simulink model "simulink_ft_fault_injection"  (R2017b)
settings: Solver=FixedStepAuto  StartTime=0.0  StopTime=Tend  FixedStep=hp  RelTol=1e-3
undefined symbols (not defined in the file): actuation_delay, Ad_plant, Bd_plant, Cd_plant, controller_mode, Dd_plant, delay_length, error_probability, f, F1, F2, F3, hp, K1, K2, K3, mode_switching_enable, n, ref, ref_array, ref_sampling_factor, Sat_u, Sm
settings Model: SimulationMode=accelerator  SnapshotInterval=2  Creator=juan  LastModifiedBy=jvalencia
settings CodeAppCC: StateflowObjectComments=on

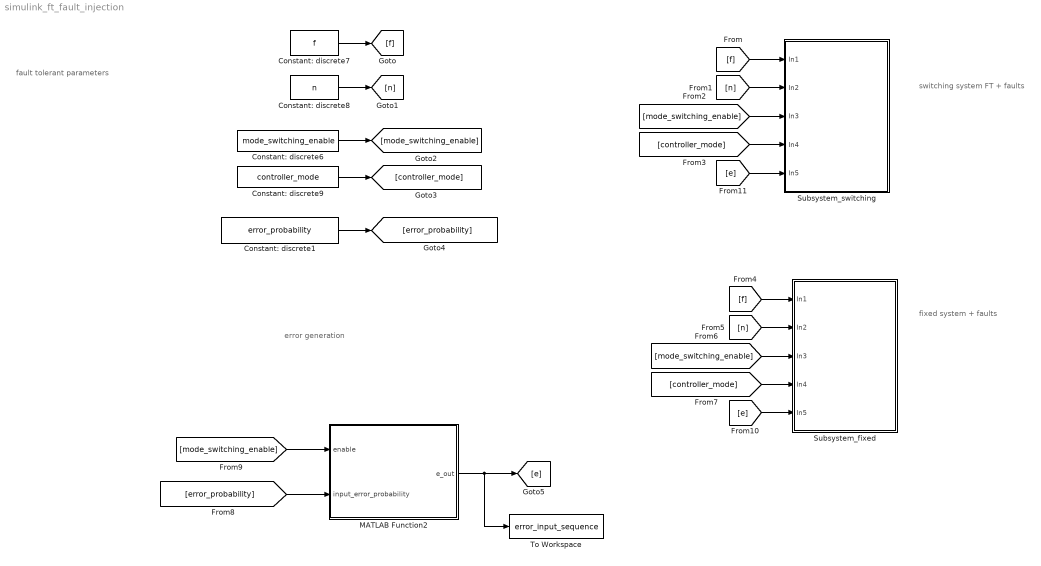
== system simulink_ft_fault_injection ==
  note: fault tolerant parameters
  note: fixed system + faults
  note: switching system FT + faults
  note: error generation
  Constant: discrete1 : Constant  Value=error_probability  SampleTime=Sm
  Constant: discrete6 : Constant  Value=mode_switching_enable  SampleTime=Sm
  Constant: discrete7 : Constant  Value=f  OutDataTypeStr=single  SampleTime=Sm
  Constant: discrete8 : Constant  Value=n  OutDataTypeStr=single  SampleTime=Sm
  Constant: discrete9 : Constant  Value=controller_mode  SampleTime=Sm
  MATLAB Function2 : MATLAB Function  TreatAsAtomicUnit=on  SystemSampleTime=Sm
  Subsystem_fixed : Subsystem
  Subsystem_switching : Subsystem
  To Workspace : ToWorkspace  VariableName=error_input_sequence  SaveFormat=Timeseries  SampleTime=Sm
  wires:
  Constant: discrete7/1 -> [f]
  Constant: discrete8/1 -> [n]
  Constant: discrete6/1 -> [mode_switching_enable]
  Constant: discrete9/1 -> [controller_mode]
  [f] -> Subsystem_switching/1(In1)
  [n] -> Subsystem_switching/2(In2)
  [mode_switching_enable] -> Subsystem_switching/3(In3)
  [controller_mode] -> Subsystem_switching/4(In4)
  Constant: discrete1/1 -> [error_probability]
  [mode_switching_enable] -> MATLAB Function2/1(enable)
  [error_probability] -> MATLAB Function2/2(input_error_probability)
  [f] -> Subsystem_fixed/1(In1)
  [n] -> Subsystem_fixed/2(In2)
  [mode_switching_enable] -> Subsystem_fixed/3(In3)
  [controller_mode] -> Subsystem_fixed/4(In4)
  MATLAB Function2/1(e_out) -> To Workspace/1, [e]
  [e] -> Subsystem_fixed/5(In5)
  [e] -> Subsystem_switching/5(In5)

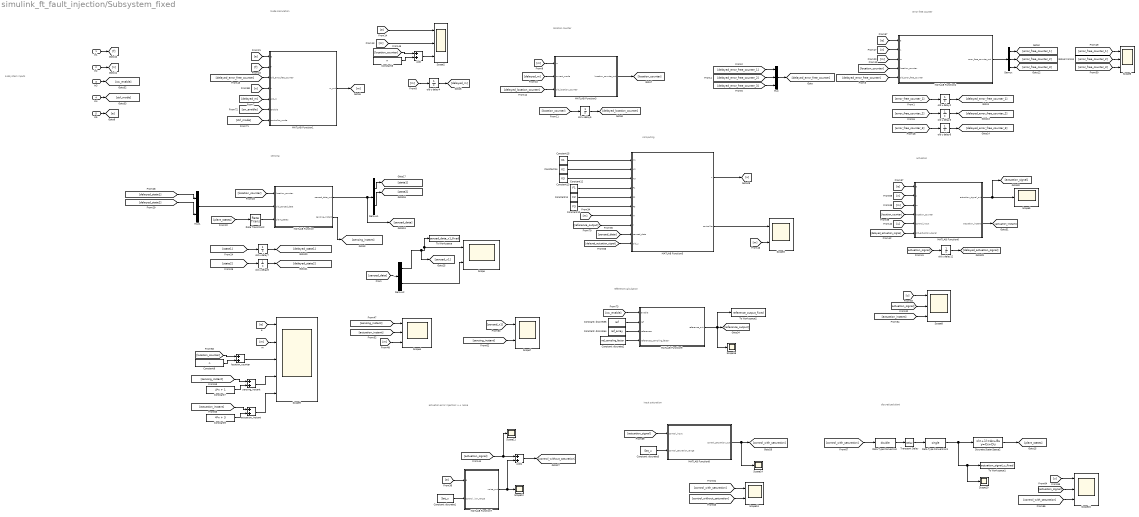
== system simulink_ft_fault_injection/Subsystem_fixed ==
  note: mode calculation
  note: location
      | counter
  note: error free counter
  note: sensing
  note: computing
  note: actuation
  note: actuation error injection: u + noise
  note: discretized plant
  note: input saturation
  note: reference calculation
  note: subsystem inputs
  In1 : Inport
  In2 : Inport  Port=2
  In3 : Inport  Port=3
  In4 : Inport  Port=4
  In5 : Inport  Port=5
  Add : Sum
  Add1 : Sum
  Constant10 : Constant  Value=F3  OutDataTypeStr=single  SampleTime=Sm
  Constant11 : Constant  Value=F2  OutDataTypeStr=single  SampleTime=Sm
  Constant12 : Constant  Value=F1  OutDataTypeStr=single  SampleTime=Sm
  Constant13 : Constant  Value=K3  OutDataTypeStr=single  SampleTime=Sm
  Constant14 : Constant  Value=K2  OutDataTypeStr=single  SampleTime=Sm
  Constant15 : Constant  Value=K1  OutDataTypeStr=single  SampleTime=Sm
  Constant6 : Constant  Value=n  SampleTime=Sm
  Constant7 : Constant  Value=4*n + 1  SampleTime=Sm
  Constant8 : Constant  Value=n  SampleTime=Sm
  Constant9 : Constant  Value=4*n + 3  SampleTime=Sm
  Constant: discrete1 : Constant  Value=Sat_u  OutDataTypeStr=single  SampleTime=Sm
  Constant: discrete2 : Constant  Value=ref_sampling_factor  OutDataTypeStr=single  SampleTime=Sm
  Constant: discrete3 : Constant  Value=Sat_u  OutDataTypeStr=single  SampleTime=Sm
  Constant: discrete4 : Constant  Value=ref_array  OutDataTypeStr=single  SampleTime=Sm
  Constant: discrete5 : Constant  Value=ref  OutDataTypeStr=single  SampleTime=Sm
  Data Type Conversion : DataTypeConversion  OutDataTypeStr=double
  Data Type Conversion1 : DataTypeConversion  OutDataTypeStr=single
  Demux : Demux  Outputs=3
  Demux1 : Demux  Outputs=2
  Demux2 : Demux  Outputs=2
  Discrete State-Space2 : DiscreteStateSpace  A=Ad_plant  B=Bd_plant  C=Cd_plant  D=Dd_plant  SampleTime=hp
  MATLAB Function : MATLAB Function  TreatAsAtomicUnit=on
  MATLAB Function1 : MATLAB Function  TreatAsAtomicUnit=on
  MATLAB Function3 : MATLAB Function  TreatAsAtomicUnit=on  SystemSampleTime=Sm
  MATLAB Function4 : MATLAB Function  TreatAsAtomicUnit=on  SystemSampleTime=Sm
  MATLAB Function5 : MATLAB Function  TreatAsAtomicUnit=on
  MATLAB Function6 : MATLAB Function  TreatAsAtomicUnit=on
  MATLAB Function7 : MATLAB Function  TreatAsAtomicUnit=on
  MATLAB Function8 : MATLAB Function  TreatAsAtomicUnit=on
  MATLAB Function9 : MATLAB Function  TreatAsAtomicUnit=on
  Mux : Mux  Inputs=3
  Mux1 : Mux  Inputs=2
  Rate Transition2 : RateTransition  OutPortSampleTime=Sm
  Scope{,3,7,13} (4 alike) : Scope  NumInputPorts=2
  Scope{5,10..12,14,16} (6 alike) : Scope
  Scope{2,4,6,8,15} (5 alike) : Scope  NumInputPorts=3
  Scope9 : Scope  NumInputPorts=5
  To Workspace : ToWorkspace  VariableName=sensed_data_x1_fixed  SaveFormat=Timeseries  SampleTime=Sm
  To Workspace1 : ToWorkspace  VariableName=actuation_signal_u_fixed  SaveFormat=Timeseries  SampleTime=Sm
  To Workspace2 : ToWorkspace  VariableName=reference_output_fixed  SaveFormat=Timeseries  SampleTime=Sm
  Transport Delay : TransportDelay  DelayTime=actuation_delay
  actuation_instant : Sum
  location_counter : Sum
  old u delay{2..8,12} (8 alike) : UnitDelay  SampleTime=Sm
  sensing_instant : Sum
  wires:
  [state2] -> old u delay8/1
  Constant14/1 -> MATLAB Function5/2(K2)
  Constant15/1 -> MATLAB Function5/1(K1)
  [reference_output] -> MATLAB Function5/8(r)
  [actuation_signal] -> Scope8/2
  [u] -> Scope8/1
  [e] -> MATLAB Function4/1(e)
  location_counter/1 -> Scope9/3
  [m] -> MATLAB Function5/7(m)
  Constant10/1 -> MATLAB Function5/6(F3)
  Constant11/1 -> MATLAB Function5/5(F2)
  Constant12/1 -> MATLAB Function5/4(F1)
  [actuation_instant] -> Scope8/3
  Demux2/1 -> [sensed_x1], To Workspace/1, Scope/1
  [e] -> MATLAB Function6/1(e)
  actuation_instant/1 -> Scope9/5
  [delayed_actuation_signal] -> MATLAB Function5/10(old_u)
  [sensed_data] -> MATLAB Function5/9(sensed_data)
  Constant13/1 -> MATLAB Function5/3(K3)
  [n] -> MATLAB Function6/2(n)
  [sensed_x1] -> Scope7/1
  Transport Delay/1 -> Data Type Conversion1/1
  [actuation_signal] -> Add1/1, Scope11/1
  MATLAB Function6/1(actuation_signal_out) -> [actuation_signal], Scope5/1
  [sensing_instant] -> Scope7/2
  Constant: discrete1/1 -> MATLAB Function7/2(control_saturation_range)
  Add1/1 -> [control_without_saturation]
  Constant: discrete3/1 -> MATLAB Function8/2(control_saturation_range)
  Data Type Conversion/1 -> Transport Delay/1
  [control_with_saturation] -> Scope13/1
  [e] -> Scope9/1
  [control_without_saturation] -> Scope13/2
  MATLAB Function8/1(control_saturation_out) -> Scope14/1, [control_with_saturation]
  [actuation_signal] -> Scope15/2
  [u] -> Scope15/1
  [control_with_saturation] -> Scope15/3
  [actuation_signal] -> MATLAB Function8/1(control_input)
  [control_with_saturation] -> Data Type Conversion/1
  [sw_enable] -> MATLAB Function1/6(enable)
  Constant: discrete4/1 -> MATLAB Function9/3(references)
  Constant: discrete5/1 -> MATLAB Function9/2(ref)
  [sw_enable] -> MATLAB Function9/1(enable)
  Constant: discrete2/1 -> MATLAB Function9/4(references_sampling_factor)
  MATLAB Function9/1(reference_out) -> To Workspace2/1, Scope16/1, [reference_output]
  Data Type Conversion1/1 -> Discrete State-Space2/1, Scope10/1, To Workspace1/1
  MATLAB Function7/1(noise_out) -> Scope12/1, Add1/2
  [e] -> MATLAB Function7/1(e)
  old u delay8/1 -> [delayed_state2]
  [state1] -> old u delay7/1
  [location_counter] -> MATLAB Function6/4(location_counter)
  Demux2/2 -> Scope/2
  [e] -> MATLAB Function1/1(e)
  [delayed_error_free_counter] -> MATLAB Function4/5(old_error_free_counter)
  [delayed_error_free_counter] -> MATLAB Function1/3(old_error_free_counter)
  Mux/1 -> [delayed_error_free_counter]
  MATLAB Function5/1(u) -> [u]
  [error_free_counter_3] -> Scope6/3
  Constant7/1 -> sensing_instant/2
  MATLAB Function5/2(controller) -> Scope3/1
  [actuation_instant] -> actuation_instant/1
  [location_counter] -> location_counter/1
  Constant9/1 -> actuation_instant/2
  [sensing_instant] -> sensing_instant/1
  [actuation_instant] -> Scope4/2
  [m] -> Scope4/3
  MATLAB Function6/2(actuation_instant) -> [actuation_instant]
  Constant8/1 -> location_counter/2
  [sensing_instant] -> Scope4/1
  [m] -> Scope9/2
  MATLAB Function/2(sensing_instant) -> [sensing_instant]
  [m] -> Scope3/2
  [error_free_counter_2] -> Scope6/2
  [error_free_counter_1] -> Scope6/1
  Add/1 -> Scope2/3
  Constant6/1 -> Add/2
  [location_counter] -> Add/1
  [delayed_state2] -> Mux1/2
  [actuation_signal] -> old u delay12/1
  [delayed_state1] -> Mux1/1
  old u delay12/1 -> [delayed_actuation_signal]
  [delayed_actuation_signal] -> MATLAB Function6/6(old_actuation_signal)
  [sensed_data] -> Demux2/1
  sensing_instant/1 -> Scope9/4
  Mux1/1 -> MATLAB Function/2(old_sensed_data)
  old u delay7/1 -> [delayed_state1]
  Rate Transition2/1 -> MATLAB Function/3(plant_states)
  [m] -> MATLAB Function6/3(m)
  [u] -> MATLAB Function6/5(control_input)
  old u delay2/1 -> [delayed_error_free_counter_1]
  [location_counter] -> old u delay5/1
  [plant_states] -> Rate Transition2/1
  [delayed_error_free_counter_3] -> Mux/3
  [m] -> MATLAB Function3/1(m)
  [n] -> MATLAB Function4/2(n)
  Demux/3 -> [error_free_counter_3]
  old u delay4/1 -> [delayed_m]
  [error_free_counter_1] -> old u delay2/1
  MATLAB Function1/1(m_out) -> [m]
  old u delay3/1 -> [delayed_error_free_counter_2]
  old u delay6/1 -> [delayed_error_free_counter_3]
  MATLAB Function/1(sensed_data_out) -> [sensed_data], Demux1/1
  Demux1/2 -> [state2]
  [delayed_error_free_counter_1] -> Mux/1
  [m] -> MATLAB Function4/3(m)
  Discrete State-Space2/1 -> [plant_states]
  Demux/2 -> [error_free_counter_2]
  [delayed_error_free_counter_2] -> Mux/2
  [delayed_m] -> MATLAB Function3/2(current_mode)
  MATLAB Function3/1(location_counter_out) -> [location_counter]
  [delayed_location_counter] -> MATLAB Function3/3(old_location_counter)
  old u delay5/1 -> [delayed_location_counter]
  Demux/1 -> [error_free_counter_1]
  Demux1/1 -> [state1]
  [m] -> old u delay4/1
  [location_counter] -> MATLAB Function4/4(location_counter)
  [e] -> Scope2/1
  [m] -> Scope2/2
  [error_free_counter_2] -> old u delay3/1
  [delayed_m] -> MATLAB Function1/5(old_m)
  [error_free_counter_3] -> old u delay6/1
  MATLAB Function4/1(error_free_counter_out) -> Demux/1
  [location_counter] -> MATLAB Function/1(location_counter)
  [ctrl_mode] -> MATLAB Function1/7(controller_mode)
  [f] -> MATLAB Function1/2(f)
  [n] -> MATLAB Function1/4(n)
  In1/1 -> [f]
  In2/1 -> [n]
  In3/1 -> [sw_enable]
  In4/1 -> [ctrl_mode]
  In5/1 -> [e]

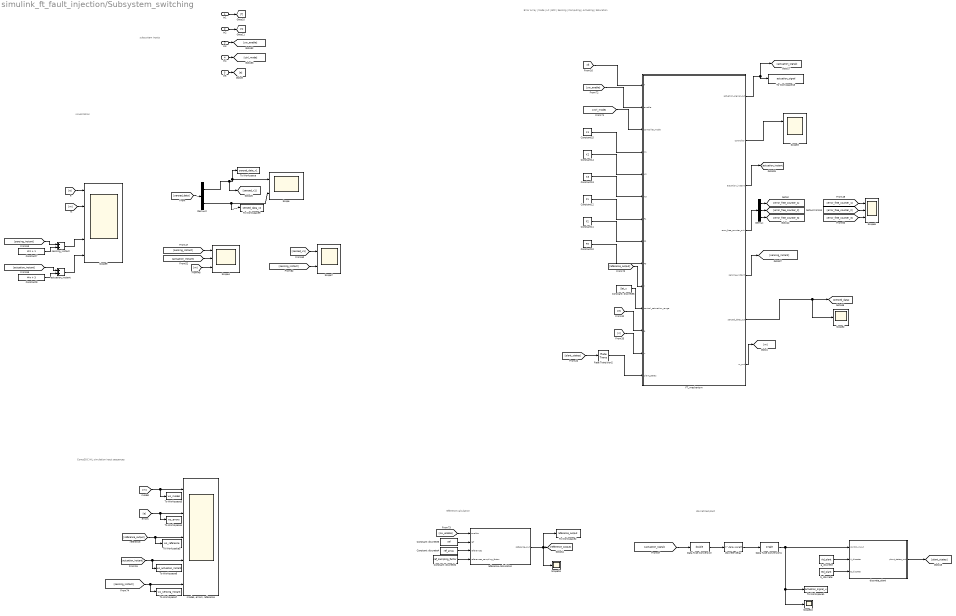
== system simulink_ft_fault_injection/Subsystem_switching ==
  note: Error Array | Mode | LC | EFC |
      | Sensing | Computing | Actuating | Saturation
  note: discretized plant
  note: reference calculation
  note: subsystem inputs
  note: CompSOC HIL simulation input sequences
  note: visualization
  In1 : Inport
  In2 : Inport  Port=2
  In3 : Inport  Port=3
  In4 : Inport  Port=4
  In5 : Inport  Port=5
  Constant10 : Constant  Value=F3  OutDataTypeStr=single  SampleTime=Sm
  Constant11 : Constant  Value=F2  OutDataTypeStr=single  SampleTime=Sm
  Constant12 : Constant  Value=F1  OutDataTypeStr=single  SampleTime=Sm
  Constant13 : Constant  Value=K3  OutDataTypeStr=single  SampleTime=Sm
  Constant14 : Constant  Value=K2  OutDataTypeStr=single  SampleTime=Sm
  Constant15 : Constant  Value=K1  OutDataTypeStr=single  SampleTime=Sm
  Constant7 : Constant  Value=4*n + 1  SampleTime=Sm
  Constant9 : Constant  Value=4*n + 3  SampleTime=Sm
  Constant: discrete2 : Constant  Value=ref_sampling_factor  OutDataTypeStr=single  SampleTime=Sm
  Constant: discrete4 : Constant  Value=ref_array  OutDataTypeStr=single  SampleTime=Sm
  Constant: discrete5 : Constant  Value=ref  OutDataTypeStr=single  SampleTime=Sm
  Constant: discrete6 : Constant  Value=Sat_u  OutDataTypeStr=single  SampleTime=Sm
  Data Type Conversion : DataTypeConversion  OutDataTypeStr=double
  Data Type Conversion1 : DataTypeConversion  OutDataTypeStr=single
  Demux : Demux  Outputs=3
  Demux2 : Demux  Outputs=2
  FT_mechanism : MATLAB Function  TreatAsAtomicUnit=on
  Rate Transition2 : RateTransition  OutPortSampleTime=Sm
  Scope : Scope  NumInputPorts=2
  Scope10 : Scope
  Scope16 : Scope
  Scope2 : Scope
  Scope3 : Scope  NumInputPorts=2
  Scope4 : Scope  NumInputPorts=3
  Scope6 : Scope  NumInputPorts=3
  Scope7 : Scope  NumInputPorts=2
  Scope9 : Scope  NumInputPorts=5
  To Workspace : ToWorkspace  VariableName=sensed_data_x1  SaveFormat=Timeseries  SampleTime=Sm
  To Workspace1 : ToWorkspace  VariableName=actuation_signal_u  SaveFormat=Timeseries  SampleTime=Sm
  To Workspace13 : ToWorkspace  VariableName=actuation_signal  SaveFormat=Timeseries  SampleTime=Sm
  To Workspace2 : ToWorkspace  VariableName=reference_output  SaveFormat=Timeseries  SampleTime=Sm
  To Workspace3 : ToWorkspace  VariableName=ws_modes  SaveFormat=Timeseries  SampleTime=Sm
  To Workspace4 : ToWorkspace  VariableName=ws_errors  SaveFormat=Timeseries  SampleTime=Sm
  To Workspace5 : ToWorkspace  VariableName=ws_reference  SaveFormat=Timeseries  SampleTime=Sm
  To Workspace6 : ToWorkspace  VariableName=ws_actuation_instant  SaveFormat=Timeseries  SampleTime=Sm
  To Workspace7 : ToWorkspace  VariableName=ws_sensing_instant  SaveFormat=Timeseries  SampleTime=Sm
  To Workspace9 : ToWorkspace  VariableName=sensed_data_x2  SaveFormat=Timeseries  SampleTime=Sm
  a_discrete : Constant  Value=Ad_plant  OutDataTypeStr=single  SampleTime=hp
  actuation_instant : Sum
  b_discrete : Constant  Value=Bd_plant  OutDataTypeStr=single  SampleTime=hp
  discrete-delay : Delay  DelayLength=delay_length  SampleTime=hp
  discrete_plant : MATLAB Function  TreatAsAtomicUnit=on  SystemSampleTime=hp
  "modes, errors, reference" : Scope  NumInputPorts=5
  reference-calculation : MATLAB Function  TreatAsAtomicUnit=on
  sensing_instant : Sum
  wires:
  Constant14/1 -> FT_mechanism/5(K2)
  Constant15/1 -> FT_mechanism/4(K1)
  [reference_output] -> FT_mechanism/10(r)
  Constant10/1 -> FT_mechanism/9(F3)
  Constant11/1 -> FT_mechanism/8(F2)
  Constant12/1 -> FT_mechanism/7(F1)
  Demux2/1 -> [sensed_x1], To Workspace/1, Scope/1
  actuation_instant/1 -> Scope9/5
  Constant13/1 -> FT_mechanism/6(K3)
  [sensed_x1] -> Scope7/1
  discrete-delay/1 -> Data Type Conversion1/1
  [sensing_instant] -> Scope7/2
  Data Type Conversion/1 -> discrete-delay/1
  [e] -> Scope9/1
  [actuation_signal] -> Data Type Conversion/1
  Constant: discrete4/1 -> reference-calculation/3(references)
  Constant: discrete5/1 -> reference-calculation/2(ref)
  [sw_enable] -> reference-calculation/1(enable)
  Constant: discrete2/1 -> reference-calculation/4(references_sampling_factor)
  reference-calculation/1(reference_out) -> To Workspace2/1, Scope16/1, [reference_output]
  Data Type Conversion1/1 -> discrete_plant/1(control_input), To Workspace1/1, Scope10/1
  Demux2/2 -> To Workspace9/1, Scope/2
  FT_mechanism/1(actuation_signal_out) -> To Workspace13/1, [actuation_signal]
  [error_free_counter_3] -> Scope6/3
  Constant7/1 -> sensing_instant/2
  FT_mechanism/2(controller) -> Scope3/1
  [actuation_instant] -> actuation_instant/1
  Constant9/1 -> actuation_instant/2
  [sensing_instant] -> sensing_instant/1
  [actuation_instant] -> Scope4/2
  [m] -> Scope4/3
  [sensing_instant] -> Scope4/1
  [m] -> Scope9/2
  [error_free_counter_2] -> Scope6/2
  [error_free_counter_1] -> Scope6/1
  [sensed_data] -> Demux2/1
  sensing_instant/1 -> Scope9/4
  In1/1 -> [f]
  In2/1 -> [n]
  In3/1 -> [sw_enable]
  In4/1 -> [ctrl_mode]
  In5/1 -> [e]
  [m] -> To Workspace3/1, "modes, errors, reference"/1
  [reference_output] -> "modes, errors, reference"/3, To Workspace5/1
  [e] -> To Workspace4/1, "modes, errors, reference"/2
  [actuation_instant] -> To Workspace6/1, "modes, errors, reference"/4
  [sensing_instant] -> To Workspace7/1, "modes, errors, reference"/5
  a_discrete/1 -> discrete_plant/2(A_discrete)
  b_discrete/1 -> discrete_plant/3(B_discrete)
  discrete_plant/1(plant_states_out) -> [plant_states]
  Constant: discrete6/1 -> FT_mechanism/11(control_saturation_range)
  FT_mechanism/3(actuation_instant) -> [actuation_instant]
  [n] -> FT_mechanism/13(n)
  [e] -> FT_mechanism/12(e)
  Demux/3 -> [error_free_counter_3]
  Demux/2 -> [error_free_counter_2]
  Demux/1 -> [error_free_counter_1]
  FT_mechanism/4(error_free_counter_out) -> Demux/1
  Rate Transition2/1 -> FT_mechanism/14(plant_states)
  [plant_states] -> Rate Transition2/1
  FT_mechanism/6(sensed_data_out) -> Scope2/1, [sensed_data]
  FT_mechanism/5(sensing_instant) -> [sensing_instant]
  [sw_enable] -> FT_mechanism/2(enable)
  [ctrl_mode] -> FT_mechanism/3(controller_mode)
  [f] -> FT_mechanism/1(f)
  FT_mechanism/7(m_out) -> [m]

== matlab function simulink_ft_fault_injection/Subsystem_switching/discrete_plant ==
  data: control_input input single; plant_states_out output single; A_discrete input single; B_discrete input single
function plant_states_out = discrete_plant(control_input, A_discrete, B_discrete)

persistent state;
if (isempty(state)) %It does not already exist
state = single(zeros(2,1)); % initialize with 0
end

plant_states_out = A_discrete*state + B_discrete*control_input;
state = single(plant_states_out);

== matlab function simulink_ft_fault_injection/Subsystem_switching/FT_mechanism ==
  data: f input; enable input; controller_mode input; K1 input single; K2 input single; K3 input; F1 input; F2 input; F3 input; r input single; control_saturation_range input; e input; n input; actuation_signal_out output single; controller output; actuation_instant output; error_free_counter_out output size=n; sensing_instant output; plant_states input single size=2; sensed_data_out output single size=2; m_out output
function [actuation_signal_out, controller, actuation_instant, error_free_counter_out, sensing_instant, sensed_data_out, m_out] = computing(f, enable, controller_mode, K1, K2, K3, F1, F2, F3, r, control_saturation_range, e, n, plant_states)
%% initialization of persistent variables
%#eml
assert(n < 10); % less than 10 modes: limit for embedded code this can be changed

% error array
persistent e_array;
if (isempty(e_array)) %It does not already exist
    e_array = zeros(1,2^n); % initialize with 0
end

% mode
persistent m;
if (isempty(m)) %It does not already exist
    m = 1; % initialize with mode 1
end

% current mode
persistent current_mode;
if (isempty(current_mode)) %It does not already exist
    current_mode = 1; % initialize with mode 1
end

% lc
persistent location_counter;
if (isempty(location_counter)) %It does not already exist
    location_counter = 0; % initialize with 0
end

persistent lc_old;
if (isempty(lc_old)) %It does not already exist
    lc_old = 0; % initialize with 0
end


% efc
persistent error_free_counter;
if (isempty(error_free_counter)) %It does not already exist
    error_free_counter = zeros(3,1); % initialize with 0. TODO: fixed 3 = n generic coding
end

% u
persistent u;
if (isempty(u)) %It does not already exist
    u = single(0); % initialize with 0.
end

persistent old_u;
if (isempty(old_u)) %It does not already exist
    old_u = single(0); % initialize with 0.
end

% actuation_signal
persistent actuation_signal;
if (isempty(actuation_signal)) %It does not already exist
    actuation_signal = single(0); % initialize with 0.
end

persistent old_actuation_signal;
if (isempty(old_actuation_signal)) %It does not already exist
    old_actuation_signal = single(0); % initialize with 0.
end



%% error array update
% updating array
for i = 1:2^n
    if ( i < 2^n )
        e_array(i) = e_array(i+1);
    else
        e_array(i) = e; 
    end
end



%% function m_out = mode_calculation(e, f, old_error_free_counter, n, old_m, enable, controller_mode)
% algorithm
if(current_mode < n)
    for i = 1:n
        if( current_mode == i )
            if( sum(e_array(2^n-2^i+1:2^n)) >= 2^i-1 )
                if( error_free_counter(i) >= f(i) )
                    m = current_mode + 1;
                else
                    m = current_mode;
                end
            else
                if( error_free_counter(i) >= f(i) )
                    if ( current_mode > 1)
                        m = current_mode - 1;
                    else
                        m = current_mode;
                    end
                else
                    m = current_mode;
                end                                    
            end            
        end
    end
else
    for i = 1:n
        if( current_mode == i )
            if( error_free_counter(i) >= f(i) )
                m = current_mode - 1;
            else
                m = current_mode;
            end    
        end
    end
end


% USING THE ENABLE SIGNAL: ASSIGNING CONSTANT MODE IF SW IS NOT ENABLED
if enable == 1
    m_out = m;
else
    m_out = controller_mode;
end


























%% function location_counter_out = location_counter_calculation(m, current_mode, old_location_counter)
if ( location_counter >= 2^current_mode )
    location_counter = 1;
else
    if ( location_counter >= 2^m )
        location_counter = 1;
    else
        location_counter = lc_old +1;
    end
end



%% function error_free_counter_out  = error_free_counter_calculation(e, n, m, location_counter, old_error_free_counter)
% main algorithm
if (location_counter >= 2^m)
    for i = 1:n
        if ( i ~= m )
            error_free_counter(i) = 0;
        else            
            if( sum(e_array(2^n-2^i+1:2^n)) < 2^i-1 )
                error_free_counter(i) = error_free_counter(i) + 1;
            else
                error_free_counter(i) = 0;
            end          
        end
    end
       
else
    for i = 1:n
        if ( i ~= m )
            error_free_counter(i) = 0;
        else
            error_free_counter(i) = error_free_counter(i);
        end
    end    

end

error_free_counter_out = error_free_counter;





%% function [sensed_data_out,sensing_instant] = sensing(location_counter, old_sensed_data, plant_states)
persistent sensed_data;
if (isempty(sensed_data)) %It does not already exist
    %sensed_data = single(zeros(4,1)); % initialize with 0. TODO: make generic 4 = dimension
    sensed_data = single(zeros(2,1)); % initialize with 0. TODO: make generic 4 = dimension
end

if ( location_counter == 1 )
    sensed_data = plant_states;
    sensing_instant = 1;
else
    %sensed_data = sensed_data;
    sensing_instant = 0;
end

sensed_data_out =  sensed_data;



%% computation
z = [sensed_data; old_u];

K1 = K1';
K2 = K2';
K3 = K3';

if ( m == 1 )
    u = K1*z + F1*r ;
    controller = 1;
elseif ( m == 2 )
    u = K2*z + F2*r ;
    controller = 2;
elseif ( m == 3 )
    u = K3*z + F3*r ;
    controller = 3;
else
    u = single(-100); % error value: to point out a possible fault
    controller = -100;
%     warning('something wrong with the control mode')
end



%% function [actuation_signal_out,actuation_instant] = actuating(e, n, m, location_counter, control_input, old_actuation_signal)
% main algorithm
if ( location_counter == 2^m )
    if( sum(e_array(2^n-2^m+1:2^n)) >= 2^m-1 )
        %actuation_signal = old_actuation_signal; % fault effect (use old sample)
        actuation_signal = single(0); % fault effect (zero the actuation signal)
    else
        actuation_signal = u;
    end        
    actuation_instant = 1;
else
    actuation_instant = 0;
end




%% saturation
% if actuation_signal <= min(control_saturation_range)
%     actuation_signal_out = min(control_saturation_range);
% elseif actuation_signal >= max(control_saturation_range)
%     actuation_signal_out = max(control_saturation_range);
% else
%     actuation_signal_out = actuation_signal;
% end

actuation_signal_out = actuation_signal;


%% update old signals
current_mode = m;
lc_old = location_counter;
old_actuation_signal = actuation_signal;
old_u = u;

== matlab function simulink_ft_fault_injection/Subsystem_switching/reference-calculation ==
  data: enable input; ref input; references input; reference_out output; references_sampling_factor input
function reference_out = input_reference(enable, ref, references, references_sampling_factor)
%% VARIABLE DECLARATIONS OF COUNTERS
persistent reference_counter;
if (isempty(reference_counter)) %It does not already exist
    reference_counter = 1; % initialize with mode 1
end

persistent sampling_counter;
if (isempty(sampling_counter)) %It does not already exist
    sampling_counter = 1; % initialize with mode 1
end

%% READING INPUT VARIABLES TEMPORALLY
ref_temp        = ref;
references_temp = references;

%% OUTPUT
if enable == 1
    reference_out = single(references_temp(reference_counter));
else
    reference_out = single(ref_temp);
end

%% updating the sampling counter
if sampling_counter == references_sampling_factor
    sampling_counter = 1;
else
    sampling_counter = sampling_counter + 1;
end

%% updating the reference counter to select a different reference
if sampling_counter == 1
    if reference_counter < length(references_temp)
        reference_counter = reference_counter + 1;
    else
        reference_counter = 1;
    end
end

== matlab function simulink_ft_fault_injection/Subsystem_fixed/MATLAB Function ==
  data: location_counter input; sensed_data_out output single size=2; old_sensed_data input single size=2; plant_states input single; sensing_instant output
function [sensed_data_out,sensing_instant] = sensing(location_counter, old_sensed_data, plant_states)

sensed_data = old_sensed_data;

%% 
if ( location_counter == 1 )
    sensed_data = plant_states;
    sensing_instant = 1;
else
%     sensed_data = sensed_data;
    sensing_instant = 0;
end

sensed_data_out = sensed_data;

== matlab function simulink_ft_fault_injection/Subsystem_fixed/MATLAB Function1 ==
  data: e input; m_out output; f input; old_error_free_counter input; n input; old_m input; enable input; controller_mode input
function m_out = mode_calculation(e, f, old_error_free_counter, n, old_m, enable, controller_mode)
%% initialization of persistent variables
% error array
%#eml
assert(n < 10); % less than 10 modes: limit for embedded code this can be changed
persistent e_array;
if (isempty(e_array)) %It does not already exist
e_array = zeros(1,2^n); % initialize with 0
end

% mode
persistent m;
if (isempty(m)) %It does not already exist
m = 1; % initialize with mode 1
end

% current mode
persistent current_mode;
if (isempty(current_mode)) %It does not already exist
    current_mode = 1; % initialize with mode 1
else
    current_mode = old_m;
end

error_free_counter = old_error_free_counter;

%% updating input variables
for i = 1:2^n
    if ( i < 2^n )
        e_array(i) = e_array(i+1);
    else
        e_array(i) = e; 
    end
end

%% algorithm
if(current_mode < n)
    for i = 1:n
        if( current_mode == i )
            if( sum(e_array(2^n-2^i+1:2^n)) >= 2^i-1 )
                m = current_mode + 1;
            else
                if( error_free_counter(i) >= f(i) )
                    if ( current_mode > 1)
                        m = current_mode - 1;
                    else
                        m = current_mode;
                    end
                else
                    m = current_mode;
                end                                    
            end            
        end
    end
else
    for i = 1:n
        if( current_mode == i )
            if( error_free_counter(i) >= f(i) )
                m = current_mode - 1;
            else
                m = current_mode;
            end    
        end
    end
end


% USING THE ENABLE SIGNAL: ASSIGNING CONSTANT MODE IF SW IS NOT ENABLED
m_out = controller_mode;

== matlab function simulink_ft_fault_injection/Subsystem_fixed/MATLAB Function3 ==
  data: m input; location_counter_out output; current_mode input; old_location_counter input
function location_counter_out = location_counter_calculation(m, current_mode, old_location_counter)

location_counter = old_location_counter;

if ( location_counter >= 2^current_mode )
    location_counter = 1;
else
    if ( location_counter >= 2^m )
        location_counter = 1;
    else
        location_counter = location_counter +1;
    end
end

location_counter_out = location_counter;

== matlab function simulink_ft_fault_injection/Subsystem_fixed/MATLAB Function4 ==
  data: e input; n input; error_free_counter_out output size=n; m input; location_counter input; old_error_free_counter input size=n
function error_free_counter_out  = error_free_counter_calculation(e, n, m, location_counter, old_error_free_counter)
%#eml
assert(n < 10); % less than 10 modes: limit for embedded code this can be changed
persistent e_array;
if (isempty(e_array)) %It does not already exist
e_array = zeros(1,2^n); % initialize with 0
end

%% updating input variables
error_free_counter = old_error_free_counter;

for i = 1:2^n
    if ( i < 2^n )
        e_array(i) = e_array(i+1);
    else
        e_array(i) = e; 
    end
end


%% main algorithm
% if (location_counter == 2^m)
if (location_counter >= 2^m)
    for i = 1:n
        if ( i ~= m )
            error_free_counter(i) = 0;
        else            
            if( sum(e_array(2^n-2^i+1:2^n)) < 2^i-1 )
                error_free_counter(i) = error_free_counter(i) + 1;
            else
                error_free_counter(i) = error_free_counter(i);
            end          
        end
    end
else
    for i = 1:n
        if ( i ~= m )
            error_free_counter(i) = 0;
        else
            error_free_counter(i) = error_free_counter(i);
        end
    end
end

error_free_counter_out = error_free_counter;

== matlab function simulink_ft_fault_injection/Subsystem_fixed/MATLAB Function5 ==
  data: K1 input single; K2 input single; K3 input; F1 input; F2 input; F3 input; m input; r input single; sensed_data input single; u output single; old_u input single; controller output
function [u,controller] = computing(K1, K2, K3, F1, F2, F3, m, r, sensed_data, old_u)

z = [sensed_data; old_u];

% K1 = K(1:5)';
% K2 = K(6:10)';
% K3 = K(11:15)';

% F1 = F(1);
% F2 = F(2);
% F3 = F(3);

K1 = K1';
K2 = K2';
K3 = K3';

if ( m == 1 )
    u = K1*z + F1*r ;
    controller = 1;
elseif ( m == 2 )
    u = K2*z + F2*r ;
    controller = 2;
elseif ( m == 3 )
    u = K3*z + F3*r ;
    controller = 3;
else
    u = single(-100); % error value: to point out a possible fault
    controller = -100;
%     warning('something wrong with the control mode')
end

== matlab function simulink_ft_fault_injection/Subsystem_fixed/MATLAB Function6 ==
  data: e input; n input; m input; actuation_signal_out output single; location_counter input; control_input input single; old_actuation_signal input single; actuation_instant output
function [actuation_signal_out,actuation_instant] = actuating(e, n, m, location_counter, control_input, old_actuation_signal)
%#eml
assert(n < 10); % less than 10 modes: limit for embedded code this can be changed
persistent e_array;
if (isempty(e_array)) %It does not already exist
e_array = zeros(1,2^n); % initialize with 0
end

%% updating input variables
actuation_signal = old_actuation_signal;

for i = 1:2^n
    if ( i < 2^n )
        e_array(i) = e_array(i+1);
    else
        e_array(i) = e; 
    end
end

%% main algorithm
if ( location_counter == 2^m )
    if( sum(e_array(2^n-2^m+1:2^n)) >= 2^m-1 )
        actuation_signal = actuation_signal; % fault effect (use old sample)
    else
        actuation_signal = control_input;
    end        
    actuation_instant = 1;
else
%     actuation_signal = actuation_signal;
    actuation_instant = 0;
end

actuation_signal_out = actuation_signal;

== matlab function simulink_ft_fault_injection/Subsystem_fixed/MATLAB Function7 ==
  data: e input; control_saturation_range input; noise_out output single
function noise_out = control_noise(e, control_saturation_range)

noise = unifrnd(min(control_saturation_range), max(control_saturation_range));

%% OUTPUT: USING e AS A SELECTION SIGNAL
if e == 1
    noise_out = single(noise);
else
    noise_out = single(0);
end

== matlab function simulink_ft_fault_injection/Subsystem_fixed/MATLAB Function8 ==
  data: control_input input; control_saturation_range input; control_saturation_out output single
function control_saturation_out = control_saturation(control_input, control_saturation_range)

% if control_input <= min(control_saturation_range)
%     control_saturation_out = min(control_saturation_range);
% elseif control_input >= max(control_saturation_range)
%     control_saturation_out = max(control_saturation_range);
% else
%     control_saturation_out = control_input;
% end

control_saturation_out = control_input;

== matlab function simulink_ft_fault_injection/Subsystem_fixed/MATLAB Function9 ==
  data: enable input; ref input; references input; reference_out output; references_sampling_factor input
function reference_out = input_reference(enable, ref, references, references_sampling_factor)
%% VARIABLE DECLARATIONS OF COUNTERS
persistent reference_counter;
if (isempty(reference_counter)) %It does not already exist
    reference_counter = 1; % initialize with mode 1
end

persistent sampling_counter;
if (isempty(sampling_counter)) %It does not already exist
    sampling_counter = 1; % initialize with mode 1
end

%% READING INPUT VARIABLES TEMPORALLY
ref_temp        = ref;
references_temp = references;

%% OUTPUT
if enable == 1
    reference_out = single(references_temp(reference_counter));
else
    reference_out = single(ref_temp);
end

%% updating the sampling counter
if sampling_counter == references_sampling_factor
    sampling_counter = 1;
else
    sampling_counter = sampling_counter + 1;
end

%% updating the reference counter to select a different reference
if sampling_counter == 1
    if reference_counter < length(references_temp)
        reference_counter = reference_counter + 1;
    else
        reference_counter = 1;
    end
end

== matlab function simulink_ft_fault_injection/MATLAB Function2 ==
  data: e_out output; enable input; input_error_probability input
function e_out = error_generation(enable, input_error_probability)

persistent execution_counter;
if (isempty(execution_counter)) %It does not already exist
execution_counter = 1; % initialize with 1
end

persistent counter;
if (isempty(counter)) %It does not already exist
counter = 1; % initialize with 1
end

%% test sequence: c1 since there are no errors
sequence = 0; 

if ( counter == length(sequence) )
    counter = 1;
else
    counter = counter + 1;
end

e = sequence(counter);


%% test random error
error_probability = input_error_probability;

if (execution_counter < 5000 )
    error_probability_temp = error_probability(1);
else
    error_probability_temp = error_probability(2);
end

temp = unifrnd(0,1);
if (temp > (1-error_probability_temp))
    e = 1;
else
    e = 0;
end


%% enable error injection in the simulation
if enable == 1
    e_out = e;
else
    e_out = 0;
end

%% increase execution counter
execution_counter = execution_counter + 1;
